simulink model "k1vispr2"  (Simulink 8.6)
settings: Solver=ode45  StartTime=0.0  StopTime=10.0  RelTol=1e-3
libraries: cdsEpicsBinIn x38, cdsEpicsOut x14, cdsBit2Word x14, cdsCDI64 x7, cdsCDO64 x7, cdsWord2Bit x6, dac x2, cdsAdcx0 x1, TYPEBP_MASTER x1, cdsParameters x1
(part 1 of 3)
settings Model: Creator=controls  LastModifiedBy=controls
settings OptimizationCC: InitFltsAndDblsToZero=on
settings DebuggingCC: FcnCallInpInsideContextMsg=UseLocalSettings  StrictBusMsg=Warning

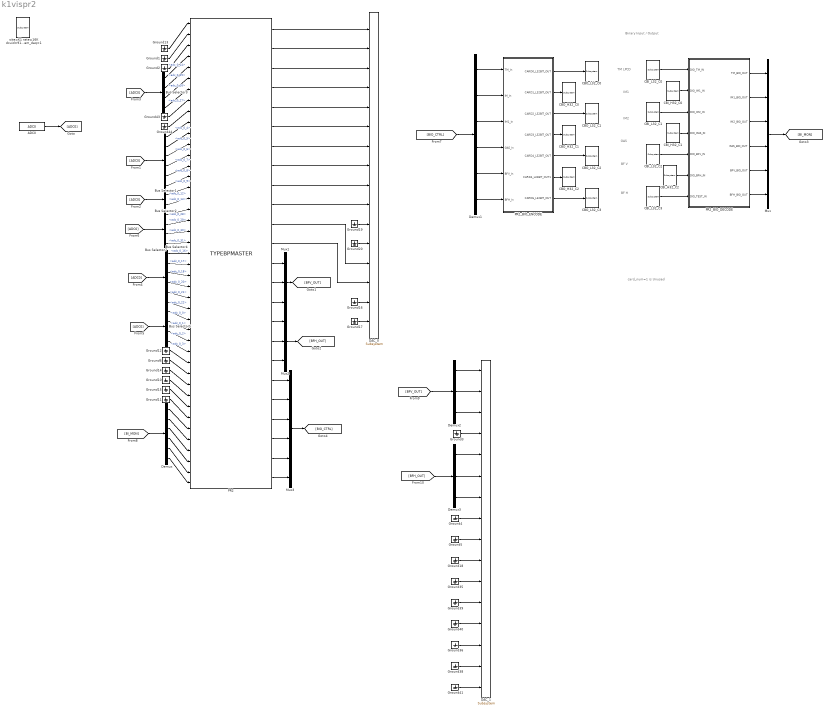
== system k1vispr2 ==
  note: TM LPCD
  note: Binary Input / Output
  note: card_num=1 is Unused
  note: IM1
  note: IM2
  note: GAS
  note: BF V
  note: BF H
  ADC0 : cdsAdcx0/ADC0  Tag=cdsAdc  Description=|
      | type-GSC_16AI64SSA
      | card_num=0
      settings: AttributesFormatString=%<Description>\n%<Tag>
  Bus Selector1 : BusSelector  Description=ADC Selector  OutputSignals=adc_0_4,adc_0_5,adc_0_6,adc_0_7,adc_0_8,adc_0_9
      settings: AttributesFormatString=%<Description>
  Bus Selector2 : BusSelector  Description=ADC Selector  OutputSignals=adc_0_12,adc_0_13
      settings: AttributesFormatString=%<Description>
  Bus Selector3 : BusSelector  Description=ADC Selector  OutputSignals=adc_0_24,adc_0_25,adc_0_26,adc_0_27
      settings: AttributesFormatString=%<Description>
  Bus Selector4 : BusSelector  Description=ADC Selector  OutputSignals=adc_0_16,adc_0_17,adc_0_18,adc_0_20,adc_0_21,adc_0_22
      settings: AttributesFormatString=%<Description>
  Bus Selector5 : BusSelector  Description=ADC Selector  OutputSignals=adc_0_0,adc_0_1,adc_0_2,adc_0_3
      settings: AttributesFormatString=%<Description>
  Bus Selector7 : BusSelector  Description=ADC Selector  OutputSignals=adc_0_28,adc_0_29,adc_0_30,adc_0_31
      settings: AttributesFormatString=%<Description>
  CBI_H32_C0 : cdsCDI64/Subsystem  Tag=cdsCDI64  Description=card_num=1
      settings: AttributesFormatString=%<Tag>\n%<Description>
  CBI_H32_C1 : cdsCDI64/Subsystem  Tag=cdsCDI64  Description=card_num=3
      settings: AttributesFormatString=%<Tag>\n%<Description>
  CBI_H32_C2 : cdsCDI64/Subsystem  Tag=cdsCDI64  Description=card_num=5
      settings: AttributesFormatString=%<Tag>\n%<Description>
  CBI_L32_C0 : cdsCDI64/Subsystem  Tag=cdsCDI64  Description=card_num=0
      settings: AttributesFormatString=%<Tag>\n%<Description>
  CBI_L32_C1 : cdsCDI64/Subsystem  Tag=cdsCDI64  Description=card_num=2
      settings: AttributesFormatString=%<Tag>\n%<Description>
  CBI_L32_C2 : cdsCDI64/Subsystem  Tag=cdsCDI64  Description=card_num=4
      settings: AttributesFormatString=%<Tag>\n%<Description>
  CBI_L32_C3 : cdsCDI64/Subsystem  Tag=cdsCDI64  Description=card_num=6
      settings: AttributesFormatString=%<Tag>\n%<Description>
  CBO_H32_C0 : cdsCDO64/Subsystem  Tag=cdsCDO64  Description=card_num=1
      settings: AttributesFormatString=%<Tag>\n%<Description>
  CBO_H32_C1 : cdsCDO64/Subsystem  Tag=cdsCDO64  Description=card_num=3
      settings: AttributesFormatString=%<Tag>\n%<Description>
  CBO_H32_C2 : cdsCDO64/Subsystem  Tag=cdsCDO64  Description=card_num=5
      settings: AttributesFormatString=%<Tag>\n%<Description>
  CBO_L32_C0 : cdsCDO64/Subsystem  Tag=cdsCDO64  Description=card_num=0
      settings: AttributesFormatString=%<Tag>\n%<Description>
  CBO_L32_C1 : cdsCDO64/Subsystem  Tag=cdsCDO64  Description=card_num=2
      settings: AttributesFormatString=%<Tag>\n%<Description>
  CBO_L32_C2 : cdsCDO64/Subsystem  Tag=cdsCDO64  Description=card_num=4
      settings: AttributesFormatString=%<Tag>\n%<Description>
  CBO_L32_C3 : cdsCDO64/Subsystem  Tag=cdsCDO64  Description=card_num=6
      settings: AttributesFormatString=%<Tag>\n%<Description>
  DAC_0 : dac/Subsystem  Description=|
      | type=GSC_16AO16,
      | card_num=0
      settings: AttributesFormatString=%<Description>
  DAC_1 : dac/Subsystem  Description=|
      | type=GSC_16AO16,
      | card_num=1
      settings: AttributesFormatString=%<Description>
  Demux : Demux  Outputs=6
  Demux1 : Demux  Outputs=6
  Demux2 : Demux  Outputs=3
  Demux3 : Demux  Outputs=3
  Ground{1..6,10..20,35..36,38..41,43..44} (25 alike) : Ground
  Mux : Mux  Inputs=6
  Mux1 : Mux  Inputs=3
  Mux2 : Mux  Inputs=3
  Mux3 : Mux  Inputs=6
  PR2 : TYPEBP_MASTER/TYPEBPMASTER  Description=TYPEBP MASTER
      settings: AttributesFormatString=%<Description>
  PR2_BIO_DECODE : Subsystem
  PR2_BIO_ENCODE : Subsystem
  site=K1 rate=16K dcuid=91 host=k1pr2 specific_cpu=3 adcSlave=1 shmem_daq=1 : cdsParameters/Subsystem  Tag=cdsParameters  Description=|
      | Purpose:                                                                                                                                                                                                                                
      | Provide system parameters to the FE code generator to properly configure the generated EPICS names, rep rate of the FE controller, and the Data Acquisition node ID for proper storage of data from this FE controller.                 
      |                                                                                                                                                                                                                                         
      | Useage:                                                                                                                                                                                                                                 
      | The part NAME field is used to identify the FE parameters. It must be of the form:                                                                                                                                                      
      | site=                                                                                                                                                                                                                                   
      | rate=                                                                                                                                                                                                                                   
      | dcuid=                                                                                                                                                                                                                                  
      |                                                                                                                                                                                                                                         
      | Where:                                                                                                                                                                                                                                  
      | site= argument may be H1, H2, L1, M1, G1, either as a single argument or multiple, for example site=H1,H2. These are the only names allowed. These will become the first two characters of all EPICS and signal names (for example G1:).
      |                                                                                                                                                                                                                                         
      | rate= may be 2K, 16K, 32K, or 64K                                                                                                                                                                                                       
      |                                                                                                                                                                                                                                         
      | dcuid= is site specific ie it must be unique at each site.
      settings: AttributesFormatString=%<Tag>
  wires:
  ADC0/1 -> [ADC0]
  Ground16/1 -> DAC_0/15
  Ground17/1 -> DAC_0/16
  Ground3/1 -> DAC_1/4
  Ground4/1 -> DAC_1/8
  Ground5/1 -> DAC_1/9
  Ground18/1 -> DAC_1/10
  Ground35/1 -> DAC_1/11
  Ground39/1 -> DAC_1/12
  Ground40/1 -> DAC_1/13
  Ground36/1 -> DAC_1/14
  Ground38/1 -> DAC_1/15
  Ground41/1 -> DAC_1/16
  PR2/1 -> DAC_0/1
  PR2/2 -> DAC_0/2
  PR2/3 -> DAC_0/3
  PR2/4 -> DAC_0/4
  PR2/5 -> DAC_0/5
  PR2/6 -> DAC_0/6
  PR2/7 -> DAC_0/7
  PR2/8 -> DAC_0/8
  PR2/9 -> DAC_0/9
  Ground19/1 -> DAC_0/11
  Ground20/1 -> DAC_0/12
  [BFV_OUT] -> Demux2/1
  Demux2/1 -> DAC_1/1
  Demux2/2 -> DAC_1/2
  Demux2/3 -> DAC_1/3
  [BFH_OUT] -> Demux3/1
  Demux3/1 -> DAC_1/5
  Demux3/2 -> DAC_1/6
  Demux3/3 -> DAC_1/7
  [ADC0] -> Bus Selector1/1
  Ground43/1 -> PR2/8
  Ground2/1 -> PR2/3
  Ground44/1 -> PR2/9
  Ground1/1 -> PR2/2
  Ground13/1 -> PR2/1
  Bus Selector1/1 -> PR2/10  "<adc_0_4>"
  Bus Selector4/1 -> PR2/22  "<adc_0_16>"
  [ADC0] -> Bus Selector2/1
  Bus Selector4/6 -> PR2/27  "<adc_0_22>"
  [ADC0] -> Bus Selector7/1
  [ADC0] -> Bus Selector4/1
  [ADC0] -> Bus Selector5/1
  Bus Selector3/4 -> PR2/7  "<adc_0_27>"
  Bus Selector3/1 -> PR2/4  "<adc_0_24>"
  Bus Selector3/3 -> PR2/6  "<adc_0_26>"
  Bus Selector3/2 -> PR2/5  "<adc_0_25>"
  [ADC0] -> Bus Selector3/1
  Bus Selector1/2 -> PR2/11  "<adc_0_5>"
  Bus Selector1/3 -> PR2/12  "<adc_0_6>"
  Bus Selector1/4 -> PR2/13  "<adc_0_7>"
  Bus Selector1/5 -> PR2/14  "<adc_0_8>"
  Bus Selector1/6 -> PR2/15  "<adc_0_9>"
  Bus Selector2/1 -> PR2/16  "<adc_0_12>"
  Bus Selector2/2 -> PR2/17  "<adc_0_13>"
  Bus Selector7/1 -> PR2/18  "<adc_0_28>"
  Bus Selector7/2 -> PR2/19  "<adc_0_29>"
  Bus Selector7/3 -> PR2/20  "<adc_0_30>"
  Bus Selector7/4 -> PR2/21  "<adc_0_31>"
  Bus Selector4/2 -> PR2/23  "<adc_0_17>"
  Bus Selector4/3 -> PR2/24  "<adc_0_18>"
  Bus Selector4/4 -> PR2/25  "<adc_0_20>"
  Bus Selector4/5 -> PR2/26  "<adc_0_21>"
  Bus Selector5/1 -> PR2/28  "<adc_0_0>"
  Bus Selector5/2 -> PR2/29  "<adc_0_1>"
  Bus Selector5/3 -> PR2/30  "<adc_0_2>"
  Bus Selector5/4 -> PR2/31  "<adc_0_3>"
  [BI_MON] -> Demux/1
  Demux/1 -> PR2/38
  Demux/2 -> PR2/39
  Demux/3 -> PR2/40
  Demux/4 -> PR2/41
  Demux/5 -> PR2/42
  Demux/6 -> PR2/43
  Ground14/1 -> PR2/34
  Ground6/1 -> PR2/33
  Ground12/1 -> PR2/32
  Ground11/1 -> PR2/37
  Ground15/1 -> PR2/36
  Ground10/1 -> PR2/35
  PR2/10 -> DAC_0/10
  PR2/11 -> DAC_0/13
  PR2/12 -> DAC_0/14
  PR2/13 -> Mux1/1
  PR2/14 -> Mux1/2
  PR2/15 -> Mux1/3
  Mux1/1 -> [BFV_OUT]
  PR2/16 -> Mux2/1
  PR2/17 -> Mux2/2
  PR2/18 -> Mux2/3
  Mux2/1 -> [BFH_OUT]
  PR2/19 -> Mux3/1
  PR2/20 -> Mux3/2
  PR2/21 -> Mux3/3
  PR2/22 -> Mux3/4
  PR2/23 -> Mux3/5
  PR2/24 -> Mux3/6
  Mux3/1 -> [BIO_CTRL]
  PR2_BIO_ENCODE/1(CARD0_L32BIT_OUT) -> CBO_L32_C0/1
  CBI_L32_C0/1 -> PR2_BIO_DECODE/1(DIO_TM_IN)
  PR2_BIO_DECODE/2(IM1_BIO_OUT) -> Mux/2
  PR2_BIO_DECODE/3(IM2_BIO_OUT) -> Mux/3
  PR2_BIO_DECODE/4(GAS_BIO_OUT) -> Mux/4
  PR2_BIO_DECODE/1(TM_BIO_OUT) -> Mux/1
  Mux/1 -> [BI_MON]
  [BIO_CTRL] -> Demux1/1
  PR2_BIO_ENCODE/2(CARD1_L32BIT_OUT) -> CBO_H32_C0/1
  PR2_BIO_ENCODE/3(CARD2_L32BIT_OUT) -> CBO_L32_C1/1
  PR2_BIO_ENCODE/5(CARD4_L32BIT_OUT) -> CBO_L32_C2/1
  Demux1/1 -> PR2_BIO_ENCODE/1(TM_In)
  Demux1/2 -> PR2_BIO_ENCODE/2(IM_In)
  Demux1/3 -> PR2_BIO_ENCODE/3(IM1_In)
  Demux1/4 -> PR2_BIO_ENCODE/4(GAS_In)
  Demux1/5 -> PR2_BIO_ENCODE/5(BFV_In)
  Demux1/6 -> PR2_BIO_ENCODE/6(BFH_In)
  CBI_L32_C1/1 -> PR2_BIO_DECODE/3(DIO_IM2_IN)
  CBI_H32_C1/1 -> PR2_BIO_DECODE/4(DIO_GAS_IN)
  CBI_L32_C2/1 -> PR2_BIO_DECODE/5(DIO_BFV_IN)
  PR2_BIO_DECODE/5(BFV_BIO_OUT) -> Mux/5
  PR2_BIO_DECODE/6(BFH_BIO_OUT) -> Mux/6
  CBI_H32_C0/1 -> PR2_BIO_DECODE/2(DIO_IM1_IN)
  PR2_BIO_ENCODE/4(CARD3_L32BIT_OUT) -> CBO_H32_C1/1
  PR2_BIO_ENCODE/6(CARD4_L32BIT_OUT1) -> CBO_H32_C2/1
  CBI_H32_C2/1 -> PR2_BIO_DECODE/6(DIO_BFH_IN)
  PR2_BIO_ENCODE/7(CARD6_L32BIT_OUT) -> CBO_L32_C3/1
  CBI_L32_C3/1 -> PR2_BIO_DECODE/7(DIO_TEST_IN)

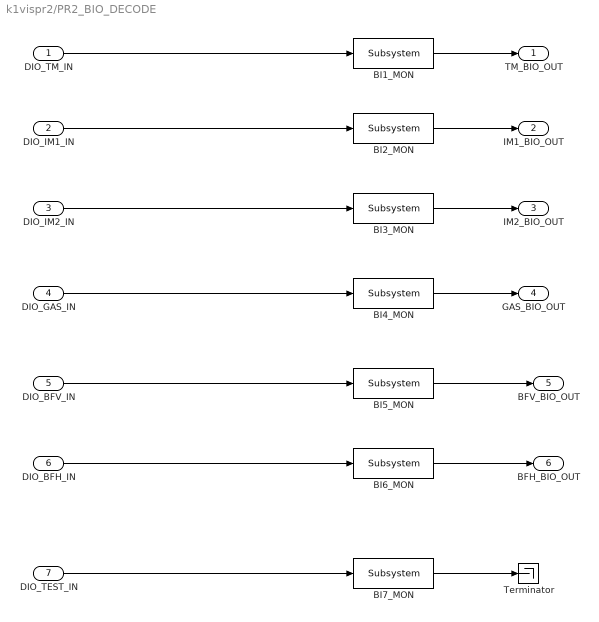
== system k1vispr2/PR2_BIO_DECODE ==
  DIO_TM_IN : Inport
  DIO_IM1_IN : Inport  Port=2
  DIO_IM2_IN : Inport  Port=3
  DIO_GAS_IN : Inport  Port=4
  DIO_BFV_IN : Inport  Port=5
  DIO_BFH_IN : Inport  Port=6
  DIO_TEST_IN : Inport  Port=7
  BI1_MON : cdsEpicsOut/Subsystem  Tag=cdsEpicsOutput  Description=|
      | Purpose:                                          
      | Output a FE signal to an EPICS channel.           
      |                                                   
      | Operation:                                        
      | Takes input value and passes it to EPICS record.  
      |                                                   
      | Usage:                                            
      | Name the part with the desired EPICS rrecord name.
      settings: AttributesFormatString=%<Tag>
  BI2_MON : cdsEpicsOut/Subsystem  Tag=cdsEpicsOutput  Description=|
      | Purpose:                                          
      | Output a FE signal to an EPICS channel.           
      |                                                   
      | Operation:                                        
      | Takes input value and passes it to EPICS record.  
      |                                                   
      | Usage:                                            
      | Name the part with the desired EPICS rrecord name.
      settings: AttributesFormatString=%<Tag>
  BI3_MON : cdsEpicsOut/Subsystem  Tag=cdsEpicsOutput  Description=|
      | Purpose:                                          
      | Output a FE signal to an EPICS channel.           
      |                                                   
      | Operation:                                        
      | Takes input value and passes it to EPICS record.  
      |                                                   
      | Usage:                                            
      | Name the part with the desired EPICS rrecord name.
      settings: AttributesFormatString=%<Tag>
  BI4_MON : cdsEpicsOut/Subsystem  Tag=cdsEpicsOutput  Description=|
      | Purpose:                                          
      | Output a FE signal to an EPICS channel.           
      |                                                   
      | Operation:                                        
      | Takes input value and passes it to EPICS record.  
      |                                                   
      | Usage:                                            
      | Name the part with the desired EPICS rrecord name.
      settings: AttributesFormatString=%<Tag>
  BI5_MON : cdsEpicsOut/Subsystem  Tag=cdsEpicsOutput  Description=|
      | Purpose:                                          
      | Output a FE signal to an EPICS channel.           
      |                                                   
      | Operation:                                        
      | Takes input value and passes it to EPICS record.  
      |                                                   
      | Usage:                                            
      | Name the part with the desired EPICS rrecord name.
      settings: AttributesFormatString=%<Tag>
  BI6_MON : cdsEpicsOut/Subsystem  Tag=cdsEpicsOutput  Description=|
      | Purpose:                                          
      | Output a FE signal to an EPICS channel.           
      |                                                   
      | Operation:                                        
      | Takes input value and passes it to EPICS record.  
      |                                                   
      | Usage:                                            
      | Name the part with the desired EPICS rrecord name.
      settings: AttributesFormatString=%<Tag>
  BI7_MON : cdsEpicsOut/Subsystem  Tag=cdsEpicsOutput  Description=|
      | Purpose:                                          
      | Output a FE signal to an EPICS channel.           
      |                                                   
      | Operation:                                        
      | Takes input value and passes it to EPICS record.  
      |                                                   
      | Usage:                                            
      | Name the part with the desired EPICS rrecord name.
      settings: AttributesFormatString=%<Tag>
  Terminator : Terminator
  TM_BIO_OUT : Outport
  IM1_BIO_OUT : Outport  Port=2
  IM2_BIO_OUT : Outport  Port=3
  GAS_BIO_OUT : Outport  Port=4
  BFV_BIO_OUT : Outport  Port=5
  BFH_BIO_OUT : Outport  Port=6
  wires:
  DIO_IM1_IN/1 -> BI2_MON/1
  DIO_TM_IN/1 -> BI1_MON/1
  DIO_IM2_IN/1 -> BI3_MON/1
  DIO_GAS_IN/1 -> BI4_MON/1
  BI1_MON/1 -> TM_BIO_OUT/1
  DIO_BFV_IN/1 -> BI5_MON/1
  BI2_MON/1 -> IM1_BIO_OUT/1
  BI3_MON/1 -> IM2_BIO_OUT/1
  BI4_MON/1 -> GAS_BIO_OUT/1
  BI5_MON/1 -> BFV_BIO_OUT/1
  DIO_BFH_IN/1 -> BI6_MON/1
  BI6_MON/1 -> BFH_BIO_OUT/1
  DIO_TEST_IN/1 -> BI7_MON/1
  BI7_MON/1 -> Terminator/1
